simulink model "project_10"  (R2020a)
settings: Solver=ode45  StartTime=0.0  StopTime=3  RelTol=1e-3
values from neighbouring files (symbols this model uses):
  b = 3.5077E-6    (= 3.5077e-06)    [project_10m.m]    (also in project_3m.m = 10; project_7m.m = 10; project_8m.m = 10; project_9m.m = 50)
  j = 3.2284E-6    (= 3.2284e-06)    [project_10m.m]
  Kb = 0.0274    [project_10m.m]
  Kt = 0.0274    [project_10m.m]
  L = 2.75E-6    (= 2.75e-06)    [project_10m.m]
  r = 4    [project_10m.m]    (also in project_9m.m = 10)
  V = 1    [project_10m.m]
libraries: simulink x1
settings Model: Creator=Matt  LastModifiedBy=Matt
settings DataIOCC: ReturnWorkspaceOutputs=off  TimeSaveName=time

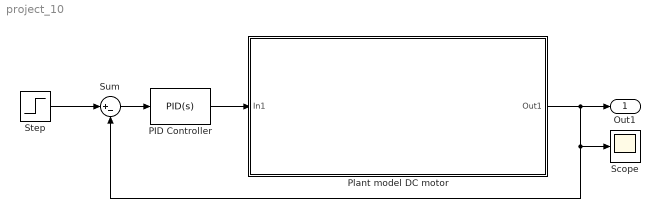
== system project_10 ==
  PID Controller : simulink/Continuous/PID Controller  Controller=PID  Form=Parallel  TimeDomain=Continuous-time  UseExternalTs=off  SampleTime=-1  IntegratorMethod=Forward Euler  FilterMethod=Forward Euler  ControllerParametersSource=internal  P=53.4267746198556  I=169.45251321447  D=0.0500274810634321  UseFilter=on  N=363.560754225367  TunerSelectOption=Transfer Function Based (PID Tuner App)  InitialConditionSource=internal  InitialConditionForIntegrator=0  InitialConditionForFilter=0  DifferentiatorICPrevScaledInput=0  ExternalReset=none  TrackingMode=off  Kt=1  LimitOutput=off  UpperSaturationLimit=inf  LowerSaturationLimit=-inf  LinearizeAsGain=on  AntiWindupMode=none  Kb=1  POutMin=[]  POutMax=[]  IOutMin=[]  IOutMax=[]  DOutMin=[]  DOutMax=[]  NOutMin=[]  NOutMax=[]  SumOutMin=[]  SumOutMax=[]  SaturationOutMin=[]  SaturationOutMax=[]  PParamMin=[]  PParamMax=[]  IParamMin=[]  IParamMax=[]  DParamMin=[]  DParamMax=[]  NParamMin=[]  NParamMax=[]  KbParamMin=[]  KbParamMax=[]  KtParamMin=[]  KtParamMax=[]  KbOutMin=[]  KbOutMax=[]  KtOutMin=[]  KtOutMax=[]  IntegratorOutMin=[]  IntegratorOutMax=[]  FilterOutMin=[]  FilterOutMax=[]  SumI1OutMin=[]  SumI1OutMax=[]  SumI2OutMin=[]  SumI2OutMax=[]  SumI3OutMin=[]  SumI3OutMax=[]  SumI4OutMin=[]  SumI4OutMax=[]  SumDOutMin=[]  SumDOutMax=[]  DifferentiatorOutMin=[]  DifferentiatorOutMax=[]  FilterDiffOutCoefMin=[]  FilterDiffOutCoefMax=[]  ReciprocalOutMin=[]  ReciprocalOutMax=[]  SumDenOutMin=[]  SumDenOutMax=[]  SumNumOutMin=[]  SumNumOutMax=[]  DivideOutMin=[]  DivideOutMax=[]  UdiffTsProdOutMin=[]  UdiffTsProdOutMax=[]  NTsProdOutMin=[]  NTsProdOutMax=[]  UintegralTsProdOutMin=[]  UintegralTsProdOutMax=[]  UngainTsProdOutMin=[]  UngainTsProdOutMax=[]  IntegratorContinuousStateAttributes=''  IntegratorStateMustResolveToSignalObject=off  IntegratorRTWStateStorageClass=Auto  FilterContinuousStateAttributes=''  FilterStateMustResolveToSignalObject=off  FilterRTWStateStorageClass=Auto  ParallelPVariant=InternalParameters  IdealPVariant=Disabled  IVariant=InternalParameters  DVariant=InternalParameters  IntegratorVariant=Continuous  SatVariant=Disabled  AWVariant=Passthrough  PCopyVariant=Disabled  TRVariant=Disabled  FdbkBlocksVariant=Forward  IdealPFdbkVariant=Disabled  SatFdbkVariant=Disabled  DerivativeFilterVariant=ContFilter  NVariant=InternalParameters  NCopyVariant=Disabled  FilterICVariant=InternalICsFilter  IntegratorICVariant=InternalICs  ExternalResetVariant=Disabled  TRSumVariant=Passthrough  SumFdbkVariant=Disabled  SumVariant=Sum_PID  TsampFilterVariant=InternalTs  TsampNgainVariant=Passthrough  TsampIntegralVariant=Passthrough
  Plant model DC motor : Subsystem
  Scope : Scope
  Step : Step  After=V  SampleTime=0
  Sum : Sum  Inputs=|+-
  Out1 : Outport
  wires:
  Step/1 -> Sum/1
  PID Controller/1 -> Plant model DC motor/1(In1)
  Sum/1 -> PID Controller/1
  Plant model DC motor/1(Out1) -> Scope/1, Sum/2, Out1/1

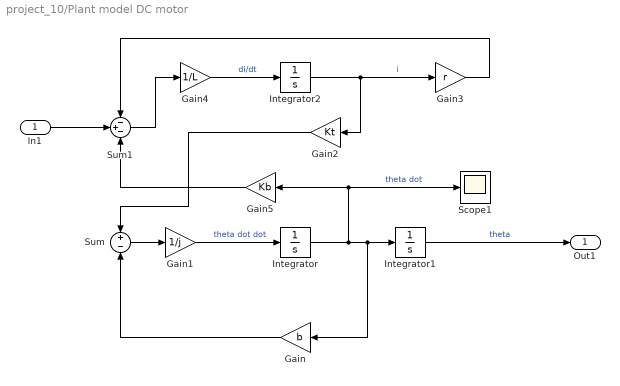
== system project_10/Plant model DC motor ==
  In1 : Inport
  Gain : Gain  Gain=b
  Gain1 : Gain  Gain=1/j
  Gain2 : Gain  Gain=Kt
  Gain3 : Gain  Gain=r
  Gain4 : Gain  Gain=1/L
  Gain5 : Gain  Gain=Kb
  Integrator : Integrator
  Integrator1 : Integrator
  Integrator2 : Integrator
  Scope1 : Scope
  Sum : Sum  Inputs=+-
  Sum1 : Sum  Inputs=-+-
  Out1 : Outport
  wires:
  Gain4/1 -> Integrator2/1  "di/dt"
  Sum/1 -> Gain1/1
  Sum1/1 -> Gain4/1
  Gain/1 -> Sum/2
  Gain3/1 -> Sum1/1
  Integrator1/1 -> Out1/1  "theta"
  Integrator2/1 -> Gain3/1, Gain2/1  "i"
  In1/1 -> Sum1/2
  Gain1/1 -> Integrator/1  "theta dot dot"
  Integrator/1 -> Scope1/1, Gain5/1, Gain/1, Integrator1/1  "theta dot"
  Gain5/1 -> Sum1/3
  Gain2/1 -> Sum/1
